simulink model "H8_2GDL_lineal_pruebas"  (R2022b)
settings: Solver=VariableStepAuto  StartTime=0.0  StopTime=5  RelTol=1e-3
InitFcn:
  | load("hems.mat");
  | airgap = hems.Airgap;
  | current = hems.Current;
  | forceV = hems.Force_Vertical;
  | forceH = hems.Force_Horizontal;
  | inductance = hems.Inductance;
  | resistance = hems.Resistance;
  | 
  | m = 200;
  | g = 9.81;
  | Iyy = 26.887;
  | x_lev12 = 0.443;
  | x_lev34 = 0.542;
  | z_max = 0.0225;
  | z_min = 0.01;
  | z_nom = 0.01965;
  | I_max = 50;
  | I_min = -50;
  | 
  | suelo = 0.0225;
  | techo = 0.01;
  | lev_nom = 0.01965;
  | time_stp = 2;
values from neighbouring files (symbols this model uses):
  A2 = argout.a    [linealizacion_2gdl.m]    (also in matrices_lineal_2gdl.mat = [0 0 689.948845287 37.4788996561 0 0 139.394129714 757.14948)
  B2 = argout.b    [linealizacion_2gdl.m]    (also in matrices_lineal_2gdl.mat = [0  0; 0  0; 0.151630617985  -0.185516467151; -0.09202917439)
  C2 = argout.c    [linealizacion_2gdl.m]    (also in matrices_lineal_2gdl.mat = [1 0 0 0 0 1 0 0 0 0 1 0 ... (16 elements, 4x4)])
  D2 = argout.d    [linealizacion_2gdl.m]    (also in matrices_lineal_2gdl.mat = [0  0; 0  0; 0  0; 0  0])
  Ka = [2091.38390024  -4523.40229407  65.4441805385  -70.1021906971  152.84626499  -886.851041867; -2276.61485995  -4503.65754193  -11.1725652788  -71.2004310761  -295.543801408  -714.324235622]    [Ka.mat]    (also in linealizacion_2gdl.m = place(Aa,Ba,[-5 -4 -6+6j -6-6j -2+2j -2-2j]))
undefined symbols (not defined in the file or in its folder): hems
libraries: slpidlib x4
settings Model: Creator=USUARIO  LastModifiedBy=ramuj

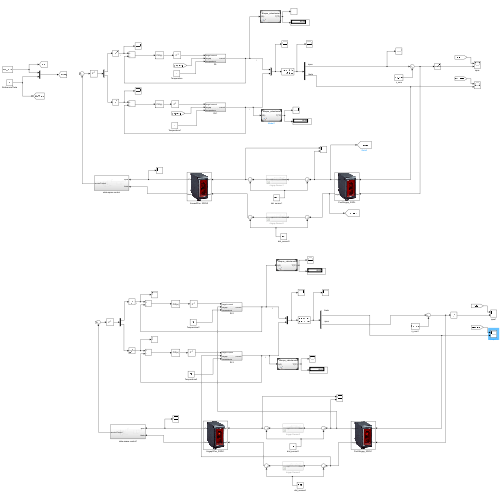
[thumbnail: Simulink's stored preview of the top-level diagram]
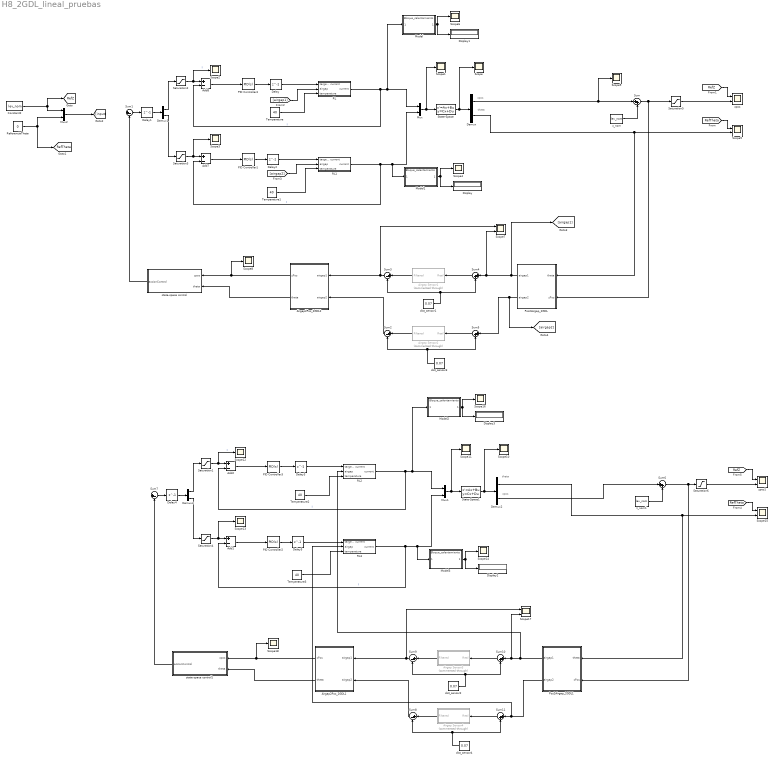
== system H8_2GDL_lineal_pruebas ==
  note: theta
  note: zpos
  note: zpos
  note: theta
  Add{1..2,7..8} (4 alike) : Sum  Inputs=+-
  Airgap Sensor1 : Subsystem  Commented=through
  Airgap Sensor2 : Subsystem  Commented=through
  Airgap Sensor3 : Subsystem  Commented=through
  Airgap Sensor4 : Subsystem  Commented=through
  Airgap2Pos_2GDL1 : Subsystem
      mask Display: image('C:\Users\ramuj\Desktop\Hyperloop\H8\Levitation-Repository\Levitation-Control-Dynamics\Modelo H8\image_airgapSensor.png'); % Use "Edit Image" on toolstrip to change.
  Airgap2Pos_2GDL2 : Subsystem
      mask Display: image('C:\Users\ramuj\Desktop\Hyperloop\H8\Levitation-Repository\Levitation-Control-Dynamics\Modelo H8\image_airgapSensor.png'); % Use "Edit Image" on toolstrip to change.
  Constant2 : Constant  Value=lev_nom
  Delay{,2..3,5} (4 alike) : Delay  DelayLength=1  SampleTime=1/(5e3)
  Delay1 : Delay  DelayLength=1  SampleTime=1/(1e3)
  Delay4 : Delay  DelayLength=1  SampleTime=1/(1e3)
  Demux{,1..3} (4 alike) : Demux  Outputs=2
  Display{,1..3} (4 alike) : Display
  Model{,1..3} (4 alike) : ModelReference  ModelNameDialog=Bloque_calentamiento.slx  SimulationMode=Normal  ModelReferenceVersion=3.3
  Mux : Mux  Inputs=2
  Mux1 : Mux  Inputs=2
  Mux2 : Mux  Inputs=2
  PID Controller{1..4} (4 alike) : slpidlib/PID Controller  Controller=PID  Form=Parallel  TimeDomain=Continuous-time  UseExternalTs=off  SampleTime=-1  IntegratorMethod=Forward Euler  FilterMethod=Forward Euler  ControllerParametersSource=internal  P=50  I=400  UseKiTs=off  D=0  N=0  UseFilter=on  TunerSelectOption=Transfer Function Based (PID Tuner App)  InitialConditionSource=internal  InitialConditionForIntegrator=0  InitialConditionForFilter=0  DifferentiatorICPrevScaledInput=0  ExternalReset=none  TrackingMode=off  Kt=1  LimitOutput=off  SatLimitsSource=internal  UpperSaturationLimit=inf  LowerSaturationLimit=-inf  LinearizeAsGain=on  AntiWindupMode=none  Kb=1  LimitIntegrator=off  UpperIntegratorSaturationLimit=inf  LowerIntegratorSaturationLimit=-inf  POutMin=[]  POutMax=[]  IOutMin=[]  IOutMax=[]  DOutMin=[]  DOutMax=[]  NOutMin=[]  NOutMax=[]  SumOutMin=[]  SumOutMax=[]  SaturationOutMin=[]  SaturationOutMax=[]  PParamMin=[]  PParamMax=[]  IParamMin=[]  IParamMax=[]  DParamMin=[]  DParamMax=[]  NParamMin=[]  NParamMax=[]  KbParamMin=[]  KbParamMax=[]  KtParamMin=[]  KtParamMax=[]  KbOutMin=[]  KbOutMax=[]  KtOutMin=[]  KtOutMax=[]  IntegratorOutMin=[]  IntegratorOutMax=[]  FilterOutMin=[]  FilterOutMax=[]  SumI1OutMin=[]  SumI1OutMax=[]  SumI2OutMin=[]  SumI2OutMax=[]  SumI3OutMin=[]  SumI3OutMax=[]  SumI4OutMin=[]  SumI4OutMax=[]  SumDOutMin=[]  SumDOutMax=[]  DifferentiatorOutMin=[]  DifferentiatorOutMax=[]  FilterDiffOutCoefMin=[]  FilterDiffOutCoefMax=[]  ReciprocalOutMin=[]  ReciprocalOutMax=[]  SumDenOutMin=[]  SumDenOutMax=[]  SumNumOutMin=[]  SumNumOutMax=[]  DivideOutMin=[]  DivideOutMax=[]  UdiffTsProdOutMin=[]  UdiffTsProdOutMax=[]  NTsProdOutMin=[]  NTsProdOutMax=[]  UintegralTsProdOutMin=[]  UintegralTsProdOutMax=[]  UngainTsProdOutMin=[]  UngainTsProdOutMax=[]  ClampingZeroOutDataTypeStr=Inherit: Inherit via back propagation  ClampingZeroOutMin=[]  ClampingZeroOutMax=[]  FilterDenConstantOutDataTypeStr=Inherit: Inherit via back propagation  FilterDenConstantOutMin=[]  FilterDenConstantOutMax=[]  PCopyOutDataTypeStr=Inherit: Inherit via back propagation  PCopyOutMin=[]  PCopyOutMax=[]  NCopyOutDataTypeStr=Inherit: Inherit via back propagation  NCopyOutMin=[]  NCopyOutMax=[]  IntegratorContinuousStateAttributes=''  IntegratorStateMustResolveToSignalObject=off  IntegratorRTWStateStorageClass=Auto  FilterContinuousStateAttributes=''  FilterStateMustResolveToSignalObject=off  FilterRTWStateStorageClass=Auto  ParallelPVariant=InternalParameters  IdealPVariant=Disabled  IVariant=InternalParameters  DVariant=InternalParameters  IntegratorVariant=Continuous  SatVariant=Disabled  AWVariant=Passthrough  PCopyVariant=Disabled  TRVariant=Disabled  FdbkBlocksVariant=Forward  IdealPFdbkVariant=Disabled  SatFdbkVariant=Disabled  DerivativeFilterVariant=ContFilter  NVariant=InternalParameters  NCopyVariant=Disabled  FilterICVariant=InternalICsFilter  IntegratorICVariant=InternalICs  ExternalResetVariant=Disabled  TRSumVariant=Passthrough  SumFdbkVariant=Disabled  SumVariant=Sum_PID  TsampFilterVariant=InternalTs  TsampNgainVariant=Passthrough  TsampIntegralVariant=Passthrough  ExternalSaturationOutDataTypeStr=Inherit: Same as second input
  Pos2Airgap_2GDL : Subsystem
      mask Display: image('C:\Users\ramuj\Desktop\Hyperloop\H8\Levitation-Repository\Levitation-Control-Dynamics\Modelo H8\image_airgapSensor.png'); % Use "Edit Image" on toolstrip to change.
  Pos2Airgap_2GDL1 : Subsystem
      mask Display: image('C:\Users\ramuj\Desktop\Hyperloop\H8\Levitation-Repository\Levitation-Control-Dynamics\Modelo H8\image_airgapSensor.png'); % Use "Edit Image" on toolstrip to change.
  RL : Subsystem
  RL1 : Subsystem
  RL2 : Subsystem
  RL3 : Subsystem
  ReferenciaTheta : Constant  Value=0
  Saturation{1..4} (4 alike) : Saturate  UpperLimit=I_max  LowerLimit=I_min
  Saturation5 : Saturate  UpperLimit=suelo  LowerLimit=techo
  Saturation6 : Saturate  UpperLimit=suelo  LowerLimit=techo
  Scope{,1..4,6,8..14,16,18} (15 alike) : Scope
  Scope{5,7,15,17} (4 alike) : Scope  NumInputPorts=2
  State-Space : StateSpace  A=A2  B=B2  C=C2  D=D2  InitialCondition=[0, suelo-lev_nom, 0, 0]
  State-Space1 : StateSpace  A=A2  B=B2  C=C2  D=D2  InitialCondition=[0, suelo-lev_nom, 0, 0]
  Sum{,4..6,10..11} (6 alike) : Sum  Inputs=|++
  Sum{1..3,7..9} (6 alike) : Sum  Inputs=|+-
  Temperature{,1..3} (4 alike) : Constant  Value=40
  dist_sensor{1..4} (4 alike) : Constant  Value=0.07
  state-space control : Subsystem
  state-space control1 : Subsystem
  z_nom : Constant  Value=lev_nom
  z_nom1 : Constant  Value=lev_nom
  zpos : Scope  NumInputPorts=2
  zpos1 : Scope  NumInputPorts=2
  tag scope: RefTheta=global, RefZ=global
  wires:
  PID Controller1/1 -> Delay2/1
  Saturation3/1 -> Scope3/1, Add7/1
  RL/1(current) -> Add8/2, Model/1, Mux/1  "I"
  PID Controller4/1 -> Delay/1
  Saturation2/1 -> Scope2/1, Add8/1  "I"
  State-Space/1 -> Demux/1, Scope/1
  Mux/1 -> Scope1/1, State-Space/1
  RL1/1(current) -> Add7/2, Mux/2, Model1/1  "I"
  z_nom/1 -> Sum/2
  Temperature/1 -> RL/3(temperature)
  Temperature1/1 -> RL1/3(temperature)
  Constant2/1 -> [RefZ], Mux2/1
  ReferenciaTheta/1 -> Mux2/2, [RefTheta]
  Mux2/1 -> [input]
  Demux1/1 -> Saturation2/1
  Demux1/2 -> Saturation3/1
  [RefTheta] -> Scope5/1
  [RefZ] -> zpos/1
  Add8/1 -> PID Controller4/1
  Add7/1 -> PID Controller1/1
  Sum1/1 -> Delay1/1
  Saturation5/1 -> zpos/2
  Model1/1 -> Scope4/1, Display/1
  Model/1 -> Scope6/1, Display1/1
  Demux/1 -> Sum/1, Scope9/1
  state-space control/1(accionControl) -> Sum1/2
  Delay1/1 -> Demux1/1
  Delay/1 -> RL/1(target current)
  Delay2/1 -> RL1/1(target current)
  Sum/1 -> Pos2Airgap_2GDL/2(zPos), Saturation5/1
  Airgap2Pos_2GDL2/1(zPos) -> Scope8/1, state-space control/1(zpos)
  Airgap2Pos_2GDL2/2(theta) -> state-space control/2(theta)
  dist_sensor1/1 -> Sum4/2, Sum3/2
  Airgap Sensor1/1(Filtered) -> Sum3/1
  Sum4/1 -> Airgap Sensor1/1(Real)
  Sum3/1 -> Scope7/1, Airgap2Pos_2GDL2/1(airgap1)
  Pos2Airgap_2GDL/1(airgap1) -> Scope7/2, Sum4/1, [airgap1]
  dist_sensor3/1 -> Sum5/2, Sum2/2
  Airgap Sensor2/1(Filtered) -> Sum2/1
  Sum5/1 -> Airgap Sensor2/1(Real)
  Pos2Airgap_2GDL/2(airgap2) -> [airgap2], Sum5/1
  Sum2/1 -> Airgap2Pos_2GDL2/2(airgap2)
  [airgap1] -> RL/2(airgap)
  [airgap2] -> RL1/2(airgap)
  Demux/2 -> Pos2Airgap_2GDL/1(theta), Scope5/2
  state-space control1/1(accionControl) -> Sum7/2
  Pos2Airgap_2GDL1/1(airgap1) -> RL2/2(airgap), Scope17/2, Sum10/1
  dist_sensor2/1 -> Sum10/2, Sum9/2
  Sum10/1 -> Airgap Sensor3/1(Real)
  Pos2Airgap_2GDL1/2(airgap2) -> RL3/2(airgap), Sum11/1
  Airgap Sensor3/1(Filtered) -> Sum9/1
  Sum6/1 -> Pos2Airgap_2GDL1/2(zPos), Saturation6/1
  Airgap2Pos_2GDL1/2(theta) -> state-space control1/2(theta)
  Sum11/1 -> Airgap Sensor4/1(Real)
  Airgap Sensor4/1(Filtered) -> Sum8/1
  dist_sensor4/1 -> Sum11/2, Sum8/2
  PID Controller2/1 -> Delay5/1
  State-Space1/1 -> Demux2/1, Scope10/1
  Temperature3/1 -> RL3/3(temperature)
  Model2/1 -> Scope16/1, Display3/1
  Demux3/2 -> Saturation4/1
  Delay3/1 -> RL2/1(target current)
  Saturation4/1 -> Scope13/1, Add1/1
  Model3/1 -> Scope14/1, Display2/1
  Delay5/1 -> RL3/1(target current)
  Sum8/1 -> Airgap2Pos_2GDL1/2(airgap2)
  Saturation6/1 -> zpos1/2
  RL2/1(current) -> Add2/2, Model2/1, Mux1/1  "I"
  Airgap2Pos_2GDL1/1(zPos) -> Scope18/1, state-space control1/1(zpos)
  Temperature2/1 -> RL2/3(temperature)
  [RefZ] -> zpos1/1
  Sum7/1 -> Delay4/1
  [RefTheta] -> Scope15/1
  Demux3/1 -> Saturation1/1
  Add2/1 -> PID Controller3/1
  Add1/1 -> PID Controller2/1
  Saturation1/1 -> Scope12/1, Add2/1  "I"
  PID Controller3/1 -> Delay3/1
  z_nom1/1 -> Sum6/2
  RL3/1(current) -> Add1/2, Mux1/2, Model3/1  "I"
  Delay4/1 -> Demux3/1
  Sum9/1 -> Scope17/1, Airgap2Pos_2GDL1/1(airgap1)
  Mux1/1 -> Scope11/1, State-Space1/1
  Demux2/1 -> Pos2Airgap_2GDL1/1(theta), Scope15/2
  Demux2/2 -> Sum6/1

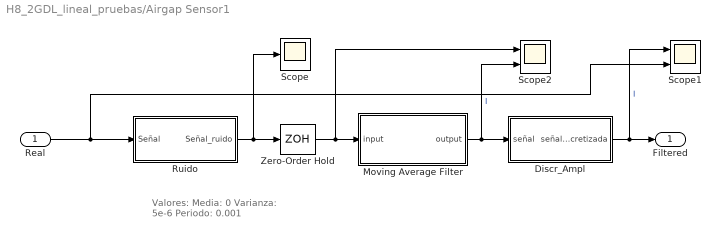
== system H8_2GDL_lineal_pruebas/Airgap Sensor1 ==
  note: Valores:
      | Media: 0
      | Varianza: 5e-6
      | Periodo: 0.001
  Real : Inport
  Discr_Ampl : Subsystem  mask{N=1024, Min=0.065, Max=0.105}
      mask prompts: N "Valores distintos (N)"; Min "Valor mínimo"; Max "Valor máximo"
      mask DialogControl DescGroupVar Prompt: Discretizacion_Amplitud
      mask DialogControl DescTextVar Prompt: Discretización en amplitud
  Moving Average Filter : Subsystem  mask{M=2, fs=-1}
      mask prompts: M "Orden del filtro (M)"; fs "Frecuencia de muestreo (fs)"
  Ruido : Subsystem  mask{M=0, V=5e-8, T=0.001}
      mask prompts: M "Media"; V "Varianza"; T "Periodo"
      mask DialogControl Ruido Prompt: Ruido
      mask DialogControl DescTextVar Prompt: Añade ruido gaussiano
  Scope : Scope
  Scope1 : Scope  NumInputPorts=2
  Scope2 : Scope  NumInputPorts=2
  Zero-Order Hold : ZeroOrderHold  SampleTime=1/(1*10^3)
  Filtered : Outport
  wires:
  Real/1 -> Scope1/2, Ruido/1(Señal)
  Discr_Ampl/1(señal_discretizada) -> Scope1/1, Filtered/1  "I"
  Moving Average Filter/1(output) -> Scope2/2, Discr_Ampl/1(señal)  "I"
  Ruido/1(Señal_ruido) -> Scope/1, Zero-Order Hold/1
  Zero-Order Hold/1 -> Moving Average Filter/1(input), Scope2/1

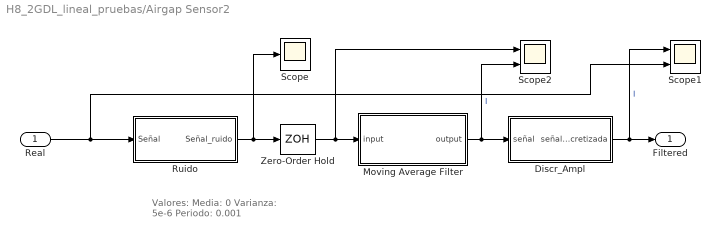
== system H8_2GDL_lineal_pruebas/Airgap Sensor2 ==
  note: Valores:
      | Media: 0
      | Varianza: 5e-6
      | Periodo: 0.001
  Real : Inport
  Discr_Ampl : Subsystem  mask{N=1024, Min=0.065, Max=0.105}
      mask prompts: N "Valores distintos (N)"; Min "Valor mínimo"; Max "Valor máximo"
      mask DialogControl DescGroupVar Prompt: Discretizacion_Amplitud
      mask DialogControl DescTextVar Prompt: Discretización en amplitud
  Moving Average Filter : Subsystem  mask{M=2, fs=-1}
      mask prompts: M "Orden del filtro (M)"; fs "Frecuencia de muestreo (fs)"
  Ruido : Subsystem  mask{M=0, V=5e-8, T=0.001}
      mask prompts: M "Media"; V "Varianza"; T "Periodo"
      mask DialogControl Ruido Prompt: Ruido
      mask DialogControl DescTextVar Prompt: Añade ruido gaussiano
  Scope : Scope
  Scope1 : Scope  NumInputPorts=2
  Scope2 : Scope  NumInputPorts=2
  Zero-Order Hold : ZeroOrderHold  SampleTime=1/(1*10^3)
  Filtered : Outport
  wires:
  Real/1 -> Scope1/2, Ruido/1(Señal)
  Discr_Ampl/1(señal_discretizada) -> Scope1/1, Filtered/1  "I"
  Moving Average Filter/1(output) -> Scope2/2, Discr_Ampl/1(señal)  "I"
  Ruido/1(Señal_ruido) -> Scope/1, Zero-Order Hold/1
  Zero-Order Hold/1 -> Moving Average Filter/1(input), Scope2/1

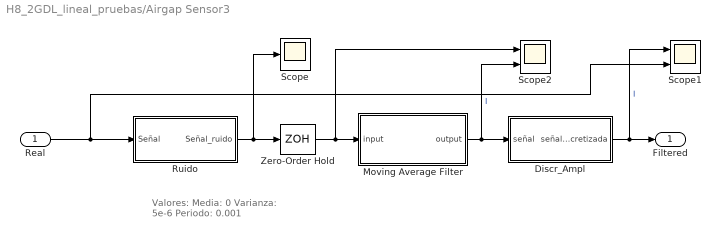
== system H8_2GDL_lineal_pruebas/Airgap Sensor3 ==
  note: Valores:
      | Media: 0
      | Varianza: 5e-6
      | Periodo: 0.001
  Real : Inport
  Discr_Ampl : Subsystem  mask{N=1024, Min=0.065, Max=0.105}
      mask prompts: N "Valores distintos (N)"; Min "Valor mínimo"; Max "Valor máximo"
      mask DialogControl DescGroupVar Prompt: Discretizacion_Amplitud
      mask DialogControl DescTextVar Prompt: Discretización en amplitud
  Moving Average Filter : Subsystem  mask{M=2, fs=-1}
      mask prompts: M "Orden del filtro (M)"; fs "Frecuencia de muestreo (fs)"
  Ruido : Subsystem  mask{M=0, V=5e-8, T=0.001}
      mask prompts: M "Media"; V "Varianza"; T "Periodo"
      mask DialogControl Ruido Prompt: Ruido
      mask DialogControl DescTextVar Prompt: Añade ruido gaussiano
  Scope : Scope
  Scope1 : Scope  NumInputPorts=2
  Scope2 : Scope  NumInputPorts=2
  Zero-Order Hold : ZeroOrderHold  SampleTime=1/(1*10^3)
  Filtered : Outport
  wires:
  Real/1 -> Scope1/2, Ruido/1(Señal)
  Discr_Ampl/1(señal_discretizada) -> Scope1/1, Filtered/1  "I"
  Moving Average Filter/1(output) -> Scope2/2, Discr_Ampl/1(señal)  "I"
  Ruido/1(Señal_ruido) -> Scope/1, Zero-Order Hold/1
  Zero-Order Hold/1 -> Moving Average Filter/1(input), Scope2/1

== system H8_2GDL_lineal_pruebas/Airgap Sensor4 ==
  note: Valores:
      | Media: 0
      | Varianza: 5e-6
      | Periodo: 0.001
  Real : Inport
  Discr_Ampl : Subsystem  mask{N=1024, Min=0.065, Max=0.105}
      mask prompts: N "Valores distintos (N)"; Min "Valor mínimo"; Max "Valor máximo"
      mask DialogControl DescGroupVar Prompt: Discretizacion_Amplitud
      mask DialogControl DescTextVar Prompt: Discretización en amplitud
  Moving Average Filter : Subsystem  mask{M=2, fs=-1}
      mask prompts: M "Orden del filtro (M)"; fs "Frecuencia de muestreo (fs)"
  Ruido : Subsystem  mask{M=0, V=5e-8, T=0.001}
      mask prompts: M "Media"; V "Varianza"; T "Periodo"
      mask DialogControl Ruido Prompt: Ruido
      mask DialogControl DescTextVar Prompt: Añade ruido gaussiano
  Scope : Scope
  Scope1 : Scope  NumInputPorts=2
  Scope2 : Scope  NumInputPorts=2
  Zero-Order Hold : ZeroOrderHold  SampleTime=1/(1*10^3)
  Filtered : Outport
  wires:
  Real/1 -> Scope1/2, Ruido/1(Señal)
  Discr_Ampl/1(señal_discretizada) -> Scope1/1, Filtered/1  "I"
  Moving Average Filter/1(output) -> Scope2/2, Discr_Ampl/1(señal)  "I"
  Ruido/1(Señal_ruido) -> Scope/1, Zero-Order Hold/1
  Zero-Order Hold/1 -> Moving Average Filter/1(input), Scope2/1

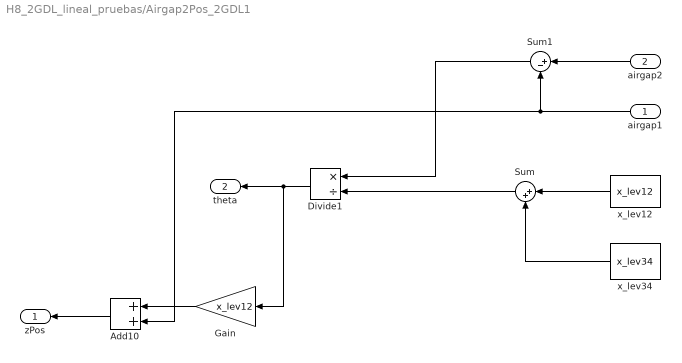
== system H8_2GDL_lineal_pruebas/Airgap2Pos_2GDL1 ==
  airgap1 : Inport
  airgap2 : Inport  Port=2
  Add10 : Sum
  Divide1 : Product  Inputs=*/
  Gain : Gain  Gain=x_lev12
  Sum : Sum  Inputs=|++
  Sum1 : Sum  Inputs=|+-
  x_lev12 : Constant  Value=x_lev12
  x_lev34 : Constant  Value=x_lev34
  zPos : Outport
  theta : Outport  Port=2
  wires:
  Add10/1 -> zPos/1
  Divide1/1 -> theta/1, Gain/1
  x_lev12/1 -> Sum/1
  x_lev34/1 -> Sum/2
  Sum/1 -> Divide1/2
  airgap2/1 -> Sum1/1
  airgap1/1 -> Sum1/2, Add10/2
  Sum1/1 -> Divide1/1
  Gain/1 -> Add10/1

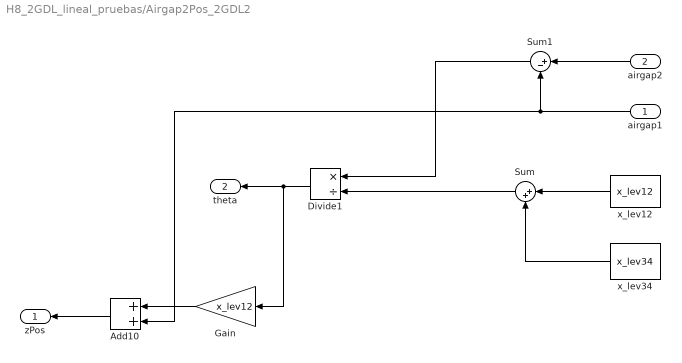
== system H8_2GDL_lineal_pruebas/Airgap2Pos_2GDL2 ==
  airgap1 : Inport
  airgap2 : Inport  Port=2
  Add10 : Sum
  Divide1 : Product  Inputs=*/
  Gain : Gain  Gain=x_lev12
  Sum : Sum  Inputs=|++
  Sum1 : Sum  Inputs=|+-
  x_lev12 : Constant  Value=x_lev12
  x_lev34 : Constant  Value=x_lev34
  zPos : Outport
  theta : Outport  Port=2
  wires:
  Add10/1 -> zPos/1
  Divide1/1 -> theta/1, Gain/1
  x_lev12/1 -> Sum/1
  x_lev34/1 -> Sum/2
  Sum/1 -> Divide1/2
  airgap2/1 -> Sum1/1
  airgap1/1 -> Sum1/2, Add10/2
  Sum1/1 -> Divide1/1
  Gain/1 -> Add10/1

== system H8_2GDL_lineal_pruebas/Pos2Airgap_2GDL ==
  theta : Inport
  zPos : Inport  Port=2
  Add10 : Sum
  Add11 : Sum  Inputs=-+
  Gain3 : Gain  Gain=x_lev12
  Gain4 : Gain  Gain=x_lev34
  airgap1 : Outport
  airgap2 : Outport  Port=2
  wires:
  Add10/1 -> airgap2/1
  zPos/1 -> Add11/2, Add10/2
  theta/1 -> Gain4/1, Gain3/1
  Gain3/1 -> Add11/1
  Gain4/1 -> Add10/1
  Add11/1 -> airgap1/1

== system H8_2GDL_lineal_pruebas/Pos2Airgap_2GDL1 ==
  theta : Inport
  zPos : Inport  Port=2
  Add10 : Sum
  Add11 : Sum  Inputs=-+
  Gain3 : Gain  Gain=x_lev12
  Gain4 : Gain  Gain=x_lev34
  airgap1 : Outport
  airgap2 : Outport  Port=2
  wires:
  Add10/1 -> airgap2/1
  zPos/1 -> Add11/2, Add10/2
  theta/1 -> Gain4/1, Gain3/1
  Gain3/1 -> Add11/1
  Gain4/1 -> Add10/1
  Add11/1 -> airgap1/1

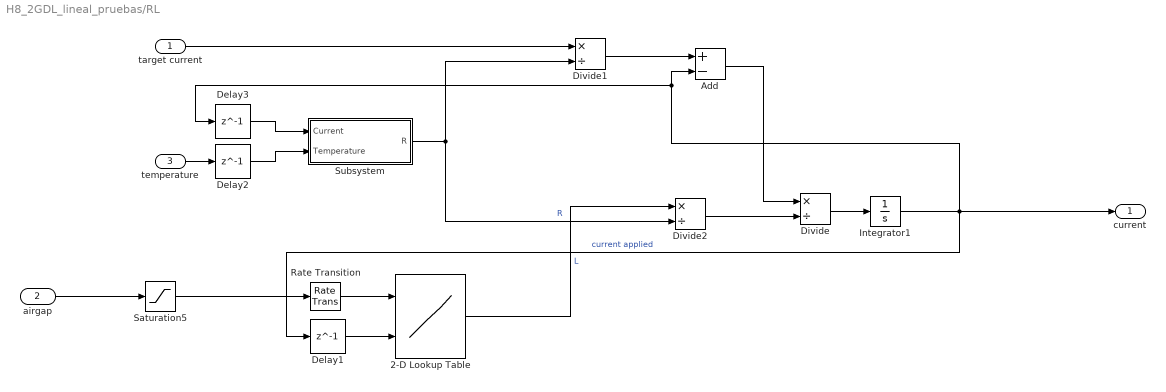
== system H8_2GDL_lineal_pruebas/RL ==
  target current : Inport
  airgap : Inport  Port=2
  temperature : Inport  Port=3
  2-D Lookup Table : Lookup_n-D  BreakpointsForDimension1=hems.Airgap  BreakpointsForDimension2=hems.Current(2:110)  Table=hems.Inductance  InternalRulePriority=Speed  RndMeth=Simplest
      settings: InputPortMap=u0,u1
  Add : Sum  Inputs=+-
  Delay1 : Delay  DelayLength=1
  Delay2 : Delay  DelayLength=1
  Delay3 : Delay  DelayLength=1
  Divide : Product  Inputs=*/
  Divide1 : Product  Inputs=*/
  Divide2 : Product  Inputs=*/
  Integrator1 : Integrator
  Rate Transition : RateTransition
  Saturation5 : Saturate  UpperLimit=suelo  LowerLimit=techo
  Subsystem : Subsystem
  current : Outport
  wires:
  airgap/1 -> Saturation5/1
  Divide/1 -> Integrator1/1
  Add/1 -> Divide/1
  Integrator1/1 -> Delay1/1, current/1, Delay3/1, Add/2  "current applied"
  2-D Lookup Table/1 -> Divide2/1  "L"
  target current/1 -> Divide1/1
  temperature/1 -> Delay2/1
  Divide1/1 -> Add/1
  Subsystem/1(R) -> Divide2/2, Divide1/2  "R"
  Delay3/1 -> Subsystem/1(Current)
  Delay2/1 -> Subsystem/2(Temperature)
  Divide2/1 -> Divide/2
  Delay1/1 -> 2-D Lookup Table/2
  Rate Transition/1 -> 2-D Lookup Table/1
  Saturation5/1 -> Rate Transition/1

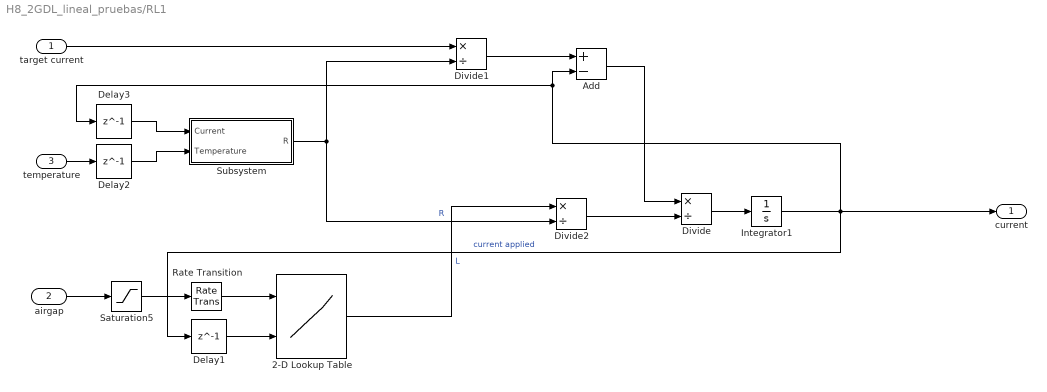
== system H8_2GDL_lineal_pruebas/RL1 ==
  target current : Inport
  airgap : Inport  Port=2
  temperature : Inport  Port=3
  2-D Lookup Table : Lookup_n-D  BreakpointsForDimension1=hems.Airgap  BreakpointsForDimension2=hems.Current(2:110)  Table=hems.Inductance  InternalRulePriority=Speed  RndMeth=Simplest
      settings: InputPortMap=u0,u1
  Add : Sum  Inputs=+-
  Delay1 : Delay  DelayLength=1
  Delay2 : Delay  DelayLength=1
  Delay3 : Delay  DelayLength=1
  Divide : Product  Inputs=*/
  Divide1 : Product  Inputs=*/
  Divide2 : Product  Inputs=*/
  Integrator1 : Integrator
  Rate Transition : RateTransition
  Saturation5 : Saturate  UpperLimit=suelo  LowerLimit=techo
  Subsystem : Subsystem
  current : Outport
  wires:
  airgap/1 -> Saturation5/1
  Divide/1 -> Integrator1/1
  Add/1 -> Divide/1
  Integrator1/1 -> Delay1/1, current/1, Delay3/1, Add/2  "current applied"
  2-D Lookup Table/1 -> Divide2/1  "L"
  target current/1 -> Divide1/1
  temperature/1 -> Delay2/1
  Divide1/1 -> Add/1
  Subsystem/1(R) -> Divide2/2, Divide1/2  "R"
  Delay3/1 -> Subsystem/1(Current)
  Delay2/1 -> Subsystem/2(Temperature)
  Divide2/1 -> Divide/2
  Delay1/1 -> 2-D Lookup Table/2
  Rate Transition/1 -> 2-D Lookup Table/1
  Saturation5/1 -> Rate Transition/1

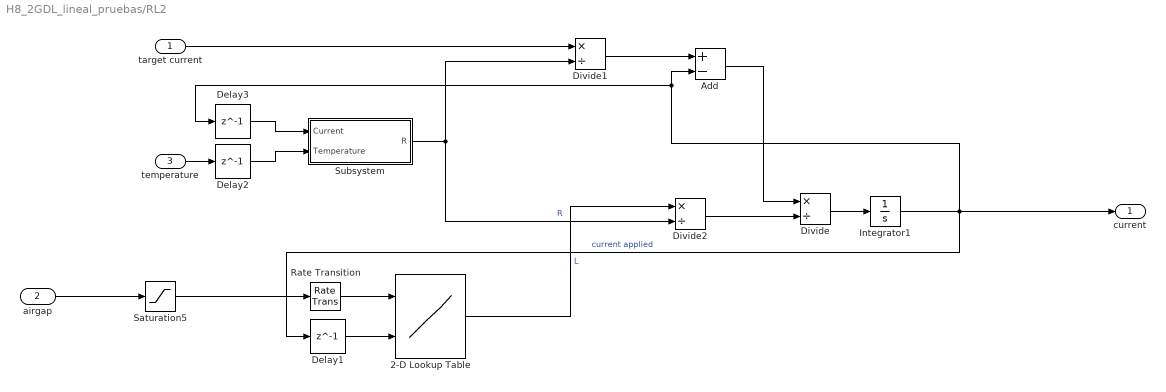
== system H8_2GDL_lineal_pruebas/RL2 ==
  target current : Inport
  airgap : Inport  Port=2
  temperature : Inport  Port=3
  2-D Lookup Table : Lookup_n-D  BreakpointsForDimension1=hems.Airgap  BreakpointsForDimension2=hems.Current(2:110)  Table=hems.Inductance  InternalRulePriority=Speed  RndMeth=Simplest
      settings: InputPortMap=u0,u1
  Add : Sum  Inputs=+-
  Delay1 : Delay  DelayLength=1
  Delay2 : Delay  DelayLength=1
  Delay3 : Delay  DelayLength=1
  Divide : Product  Inputs=*/
  Divide1 : Product  Inputs=*/
  Divide2 : Product  Inputs=*/
  Integrator1 : Integrator
  Rate Transition : RateTransition
  Saturation5 : Saturate  UpperLimit=suelo  LowerLimit=techo
  Subsystem : Subsystem
  current : Outport
  wires:
  airgap/1 -> Saturation5/1
  Divide/1 -> Integrator1/1
  Add/1 -> Divide/1
  Integrator1/1 -> Delay1/1, current/1, Delay3/1, Add/2  "current applied"
  2-D Lookup Table/1 -> Divide2/1  "L"
  target current/1 -> Divide1/1
  temperature/1 -> Delay2/1
  Divide1/1 -> Add/1
  Subsystem/1(R) -> Divide2/2, Divide1/2  "R"
  Delay3/1 -> Subsystem/1(Current)
  Delay2/1 -> Subsystem/2(Temperature)
  Divide2/1 -> Divide/2
  Delay1/1 -> 2-D Lookup Table/2
  Rate Transition/1 -> 2-D Lookup Table/1
  Saturation5/1 -> Rate Transition/1

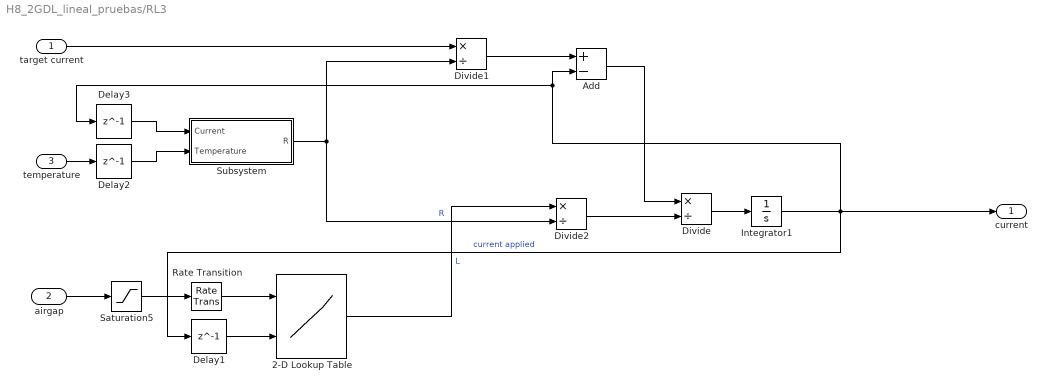
== system H8_2GDL_lineal_pruebas/RL3 ==
  target current : Inport
  airgap : Inport  Port=2
  temperature : Inport  Port=3
  2-D Lookup Table : Lookup_n-D  BreakpointsForDimension1=hems.Airgap  BreakpointsForDimension2=hems.Current(2:110)  Table=hems.Inductance  InternalRulePriority=Speed  RndMeth=Simplest
      settings: InputPortMap=u0,u1
  Add : Sum  Inputs=+-
  Delay1 : Delay  DelayLength=1
  Delay2 : Delay  DelayLength=1
  Delay3 : Delay  DelayLength=1
  Divide : Product  Inputs=*/
  Divide1 : Product  Inputs=*/
  Divide2 : Product  Inputs=*/
  Integrator1 : Integrator
  Rate Transition : RateTransition
  Saturation5 : Saturate  UpperLimit=suelo  LowerLimit=techo
  Subsystem : Subsystem
  current : Outport
  wires:
  airgap/1 -> Saturation5/1
  Divide/1 -> Integrator1/1
  Add/1 -> Divide/1
  Integrator1/1 -> Delay1/1, current/1, Delay3/1, Add/2  "current applied"
  2-D Lookup Table/1 -> Divide2/1  "L"
  target current/1 -> Divide1/1
  temperature/1 -> Delay2/1
  Divide1/1 -> Add/1
  Subsystem/1(R) -> Divide2/2, Divide1/2  "R"
  Delay3/1 -> Subsystem/1(Current)
  Delay2/1 -> Subsystem/2(Temperature)
  Divide2/1 -> Divide/2
  Delay1/1 -> 2-D Lookup Table/2
  Rate Transition/1 -> 2-D Lookup Table/1
  Saturation5/1 -> Rate Transition/1

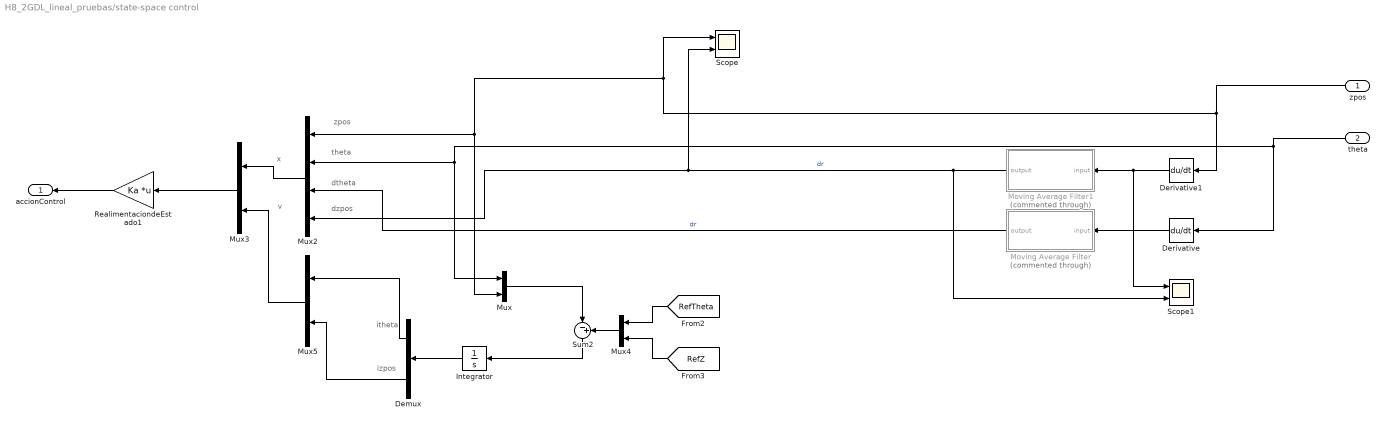
== system H8_2GDL_lineal_pruebas/state-space control ==
  note: itheta
  note: v
  note: x
  note: dtheta
  note: dzpos
  note: zpos
  note: theta
  note: izpos
  zpos : Inport
  theta : Inport  Port=2
  Demux : Demux  Outputs=2
  Derivative : Derivative
  Derivative1 : Derivative
  Integrator : Integrator
  Moving Average Filter : Subsystem  Commented=through  mask{M=2, fs=-1}
      mask prompts: M "Orden del filtro (M)"; fs "Frecuencia de muestreo (fs)"
  Moving Average Filter1 : Subsystem  Commented=through  mask{M=2, fs=-1}
      mask prompts: M "Orden del filtro (M)"; fs "Frecuencia de muestreo (fs)"
  Mux{,3..5} (4 alike) : Mux  Inputs=2
  Mux2 : Mux
  RealimentaciondeEstado1 : Gain  Gain=Ka  Multiplication=Matrix(K*u)
  Scope : Scope  NumInputPorts=2
  Scope1 : Scope  NumInputPorts=2
  Sum2 : Sum  Inputs=|-+
  accionControl : Outport
  wires:
  [RefZ] -> Mux4/2
  Derivative1/1 -> Scope1/1, Moving Average Filter1/1(input)
  zpos/1 -> Scope/1, Mux/2, Mux2/1, Derivative1/1
  Mux4/1 -> Sum2/2
  Sum2/1 -> Integrator/1
  Mux3/1 -> RealimentaciondeEstado1/1
  theta/1 -> Derivative/1, Mux2/2, Mux/1
  [RefTheta] -> Mux4/1
  Derivative/1 -> Moving Average Filter/1(input)
  RealimentaciondeEstado1/1 -> accionControl/1
  Mux/1 -> Sum2/1
  Moving Average Filter/1(output) -> Mux2/3  "dr"
  Moving Average Filter1/1(output) -> Scope1/2, Mux2/4, Scope/2  "dr"
  Mux5/1 -> Mux3/2
  Mux2/1 -> Mux3/1
  Integrator/1 -> Demux/1
  Demux/2 -> Mux5/2
  Demux/1 -> Mux5/1

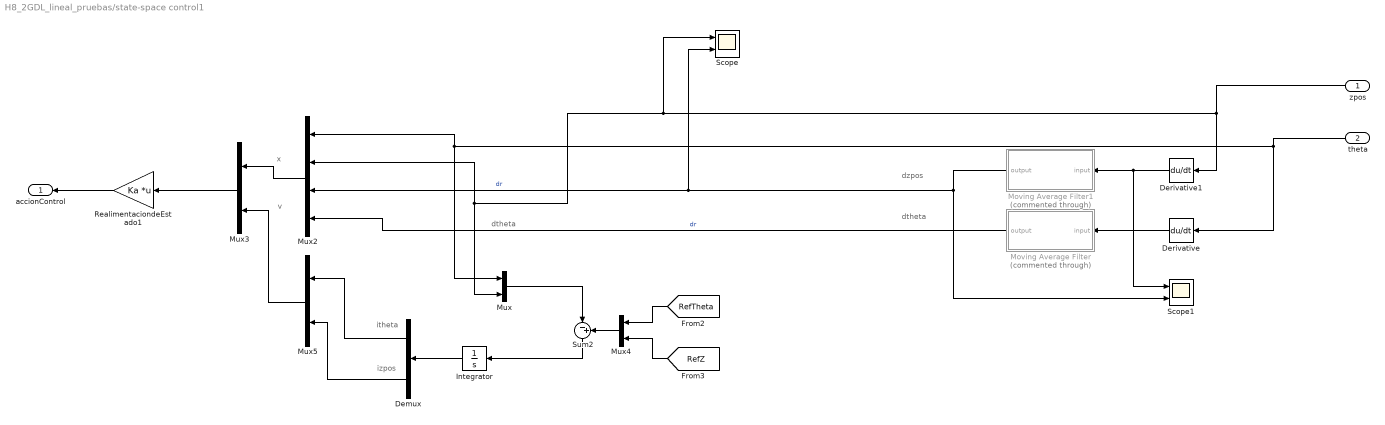
== system H8_2GDL_lineal_pruebas/state-space control1 ==
  note: dzpos
  note: itheta
  note: v
  note: x
  note: dtheta
  note: izpos
  note: dtheta
  zpos : Inport
  theta : Inport  Port=2
  Demux : Demux  Outputs=2
  Derivative : Derivative
  Derivative1 : Derivative
  Integrator : Integrator
  Moving Average Filter : Subsystem  Commented=through  mask{M=2, fs=-1}
      mask prompts: M "Orden del filtro (M)"; fs "Frecuencia de muestreo (fs)"
  Moving Average Filter1 : Subsystem  Commented=through  mask{M=2, fs=-1}
      mask prompts: M "Orden del filtro (M)"; fs "Frecuencia de muestreo (fs)"
  Mux{,3..5} (4 alike) : Mux  Inputs=2
  Mux2 : Mux
  RealimentaciondeEstado1 : Gain  Gain=Ka  Multiplication=Matrix(K*u)
  Scope : Scope  NumInputPorts=2
  Scope1 : Scope  NumInputPorts=2
  Sum2 : Sum  Inputs=|-+
  accionControl : Outport
  wires:
  [RefZ] -> Mux4/2
  Derivative1/1 -> Scope1/1, Moving Average Filter1/1(input)
  zpos/1 -> Scope/1, Mux2/2, Mux/2, Derivative1/1
  Mux4/1 -> Sum2/2
  Sum2/1 -> Integrator/1
  Mux3/1 -> RealimentaciondeEstado1/1
  theta/1 -> Derivative/1, Mux/1, Mux2/1
  [RefTheta] -> Mux4/1
  Derivative/1 -> Moving Average Filter/1(input)
  RealimentaciondeEstado1/1 -> accionControl/1
  Mux/1 -> Sum2/1
  Moving Average Filter/1(output) -> Mux2/4  "dr"
  Moving Average Filter1/1(output) -> Scope1/2, Scope/2, Mux2/3  "dr"
  Mux5/1 -> Mux3/2
  Mux2/1 -> Mux3/1
  Integrator/1 -> Demux/1
  Demux/2 -> Mux5/2
  Demux/1 -> Mux5/1

== system H8_2GDL_lineal_pruebas/Airgap Sensor1/Discr_Ampl ==
  señal : Inport
  Constant : Constant  Value=N
  Constant1 : Constant  Value=Max
  Constant2 : Constant  Value=Min
  MATLAB Function1 : MATLAB Function  TreatAsAtomicUnit=on
  señal_discretizada : Outport
  wires:
  MATLAB Function1/1(senal_discretizada) -> señal_discretizada/1
  señal/1 -> MATLAB Function1/1(senal)
  Constant1/1 -> MATLAB Function1/3(Max)
  Constant/1 -> MATLAB Function1/2(N)
  Constant2/1 -> MATLAB Function1/4(Min)

== system H8_2GDL_lineal_pruebas/Airgap Sensor1/Moving Average Filter ==
  input : Inport
  Delay : Delay  DelayLength=M  SampleTime=fs
  Delay1 : Delay  DelayLength=1  SampleTime=fs
  Gain : Gain  Gain=1/M
  Sum : Sum  Inputs=|+-
  Sum1 : Sum  Inputs=|++
  output : Outport
  wires:
  input/1 -> Delay/1, Sum/1
  Delay/1 -> Sum/2
  Sum/1 -> Sum1/1
  Sum1/1 -> Delay1/1, Gain/1
  Delay1/1 -> Sum1/2
  Gain/1 -> output/1

== system H8_2GDL_lineal_pruebas/Airgap Sensor1/Ruido ==
  Señal : Inport
  Random Number : RandomNumber  Mean=M  Variance=V  Seed=3  SampleTime=T
  Sum : Sum  Inputs=|++
  Señal_ruido : Outport
  wires:
  Random Number/1 -> Sum/2
  Señal/1 -> Sum/1
  Sum/1 -> Señal_ruido/1

== system H8_2GDL_lineal_pruebas/Airgap Sensor2/Discr_Ampl ==
  señal : Inport
  Constant : Constant  Value=N
  Constant1 : Constant  Value=Max
  Constant2 : Constant  Value=Min
  MATLAB Function1 : MATLAB Function  TreatAsAtomicUnit=on
  señal_discretizada : Outport
  wires:
  MATLAB Function1/1(senal_discretizada) -> señal_discretizada/1
  señal/1 -> MATLAB Function1/1(senal)
  Constant1/1 -> MATLAB Function1/3(Max)
  Constant/1 -> MATLAB Function1/2(N)
  Constant2/1 -> MATLAB Function1/4(Min)

== system H8_2GDL_lineal_pruebas/Airgap Sensor2/Moving Average Filter ==
  input : Inport
  Delay : Delay  DelayLength=M  SampleTime=fs
  Delay1 : Delay  DelayLength=1  SampleTime=fs
  Gain : Gain  Gain=1/M
  Sum : Sum  Inputs=|+-
  Sum1 : Sum  Inputs=|++
  output : Outport
  wires:
  input/1 -> Delay/1, Sum/1
  Delay/1 -> Sum/2
  Sum/1 -> Sum1/1
  Sum1/1 -> Delay1/1, Gain/1
  Delay1/1 -> Sum1/2
  Gain/1 -> output/1

== system H8_2GDL_lineal_pruebas/Airgap Sensor2/Ruido ==
  Señal : Inport
  Random Number : RandomNumber  Mean=M  Variance=V  Seed=3  SampleTime=T
  Sum : Sum  Inputs=|++
  Señal_ruido : Outport
  wires:
  Random Number/1 -> Sum/2
  Señal/1 -> Sum/1
  Sum/1 -> Señal_ruido/1

== system H8_2GDL_lineal_pruebas/Airgap Sensor3/Discr_Ampl ==
  señal : Inport
  Constant : Constant  Value=N
  Constant1 : Constant  Value=Max
  Constant2 : Constant  Value=Min
  MATLAB Function1 : MATLAB Function  TreatAsAtomicUnit=on
  señal_discretizada : Outport
  wires:
  MATLAB Function1/1(senal_discretizada) -> señal_discretizada/1
  señal/1 -> MATLAB Function1/1(senal)
  Constant1/1 -> MATLAB Function1/3(Max)
  Constant/1 -> MATLAB Function1/2(N)
  Constant2/1 -> MATLAB Function1/4(Min)

== system H8_2GDL_lineal_pruebas/Airgap Sensor3/Moving Average Filter ==
  input : Inport
  Delay : Delay  DelayLength=M  SampleTime=fs
  Delay1 : Delay  DelayLength=1  SampleTime=fs
  Gain : Gain  Gain=1/M
  Sum : Sum  Inputs=|+-
  Sum1 : Sum  Inputs=|++
  output : Outport
  wires:
  input/1 -> Delay/1, Sum/1
  Delay/1 -> Sum/2
  Sum/1 -> Sum1/1
  Sum1/1 -> Delay1/1, Gain/1
  Delay1/1 -> Sum1/2
  Gain/1 -> output/1

== system H8_2GDL_lineal_pruebas/Airgap Sensor3/Ruido ==
  Señal : Inport
  Random Number : RandomNumber  Mean=M  Variance=V  Seed=3  SampleTime=T
  Sum : Sum  Inputs=|++
  Señal_ruido : Outport
  wires:
  Random Number/1 -> Sum/2
  Señal/1 -> Sum/1
  Sum/1 -> Señal_ruido/1

== system H8_2GDL_lineal_pruebas/Airgap Sensor4/Discr_Ampl ==
  señal : Inport
  Constant : Constant  Value=N
  Constant1 : Constant  Value=Max
  Constant2 : Constant  Value=Min
  MATLAB Function1 : MATLAB Function  TreatAsAtomicUnit=on
  señal_discretizada : Outport
  wires:
  MATLAB Function1/1(senal_discretizada) -> señal_discretizada/1
  señal/1 -> MATLAB Function1/1(senal)
  Constant1/1 -> MATLAB Function1/3(Max)
  Constant/1 -> MATLAB Function1/2(N)
  Constant2/1 -> MATLAB Function1/4(Min)

== system H8_2GDL_lineal_pruebas/Airgap Sensor4/Moving Average Filter ==
  input : Inport
  Delay : Delay  DelayLength=M  SampleTime=fs
  Delay1 : Delay  DelayLength=1  SampleTime=fs
  Gain : Gain  Gain=1/M
  Sum : Sum  Inputs=|+-
  Sum1 : Sum  Inputs=|++
  output : Outport
  wires:
  input/1 -> Delay/1, Sum/1
  Delay/1 -> Sum/2
  Sum/1 -> Sum1/1
  Sum1/1 -> Delay1/1, Gain/1
  Delay1/1 -> Sum1/2
  Gain/1 -> output/1

== system H8_2GDL_lineal_pruebas/Airgap Sensor4/Ruido ==
  Señal : Inport
  Random Number : RandomNumber  Mean=M  Variance=V  Seed=3  SampleTime=T
  Sum : Sum  Inputs=|++
  Señal_ruido : Outport
  wires:
  Random Number/1 -> Sum/2
  Señal/1 -> Sum/1
  Sum/1 -> Señal_ruido/1

== system H8_2GDL_lineal_pruebas/RL/Subsystem ==
  Current : Inport
  Temperature : Inport  Port=2
  Resistance : Constant  Value=hems.Resistance
  R : Outport
  wires:
  Resistance/1 -> R/1

== system H8_2GDL_lineal_pruebas/RL1/Subsystem ==
  Current : Inport
  Temperature : Inport  Port=2
  Resistance : Constant  Value=hems.Resistance
  R : Outport
  wires:
  Resistance/1 -> R/1

== system H8_2GDL_lineal_pruebas/RL2/Subsystem ==
  Current : Inport
  Temperature : Inport  Port=2
  Resistance : Constant  Value=hems.Resistance
  R : Outport
  wires:
  Resistance/1 -> R/1

== system H8_2GDL_lineal_pruebas/RL3/Subsystem ==
  Current : Inport
  Temperature : Inport  Port=2
  Resistance : Constant  Value=hems.Resistance
  R : Outport
  wires:
  Resistance/1 -> R/1

== system H8_2GDL_lineal_pruebas/state-space control/Moving Average Filter ==
  input : Inport
  Delay : Delay  DelayLength=M  SampleTime=fs
  Delay1 : Delay  DelayLength=1  SampleTime=fs
  Gain : Gain  Gain=1/M
  Sum : Sum  Inputs=|+-
  Sum1 : Sum  Inputs=|++
  output : Outport
  wires:
  input/1 -> Delay/1, Sum/1
  Delay/1 -> Sum/2
  Sum/1 -> Sum1/1
  Sum1/1 -> Delay1/1, Gain/1
  Delay1/1 -> Sum1/2
  Gain/1 -> output/1

== system H8_2GDL_lineal_pruebas/state-space control/Moving Average Filter1 ==
  input : Inport
  Delay : Delay  DelayLength=M  SampleTime=fs
  Delay1 : Delay  DelayLength=1  SampleTime=fs
  Gain : Gain  Gain=1/M
  Sum : Sum  Inputs=|+-
  Sum1 : Sum  Inputs=|++
  output : Outport
  wires:
  input/1 -> Delay/1, Sum/1
  Delay/1 -> Sum/2
  Sum/1 -> Sum1/1
  Sum1/1 -> Delay1/1, Gain/1
  Delay1/1 -> Sum1/2
  Gain/1 -> output/1

== system H8_2GDL_lineal_pruebas/state-space control1/Moving Average Filter ==
  input : Inport
  Delay : Delay  DelayLength=M  SampleTime=fs
  Delay1 : Delay  DelayLength=1  SampleTime=fs
  Gain : Gain  Gain=1/M
  Sum : Sum  Inputs=|+-
  Sum1 : Sum  Inputs=|++
  output : Outport
  wires:
  input/1 -> Delay/1, Sum/1
  Delay/1 -> Sum/2
  Sum/1 -> Sum1/1
  Sum1/1 -> Delay1/1, Gain/1
  Delay1/1 -> Sum1/2
  Gain/1 -> output/1

== system H8_2GDL_lineal_pruebas/state-space control1/Moving Average Filter1 ==
  input : Inport
  Delay : Delay  DelayLength=M  SampleTime=fs
  Delay1 : Delay  DelayLength=1  SampleTime=fs
  Gain : Gain  Gain=1/M
  Sum : Sum  Inputs=|+-
  Sum1 : Sum  Inputs=|++
  output : Outport
  wires:
  input/1 -> Delay/1, Sum/1
  Delay/1 -> Sum/2
  Sum/1 -> Sum1/1
  Sum1/1 -> Delay1/1, Gain/1
  Delay1/1 -> Sum1/2
  Gain/1 -> output/1

== matlab function H8_2GDL_lineal_pruebas/Airgap Sensor1/Discr_Ampl/MATLAB Function1 ==
  data: senal input; senal_discretizada output; N input; Max input; Min input
function senal_discretizada  = fcn(senal,N,Max,Min)

if(senal>Max)
    senal_discretizada=Max;
    return
elseif(senal<Min)
    senal_discretizada=Min;
    return
end

valor_escalon=(Max-Min)/(N-1);
i=Min;
 while(i<Max)
    if(i+valor_escalon/2>senal)
        senal_discretizada=i;
        return
    end
    i=i+valor_escalon;
end

      senal_discretizada=Max;
end

== matlab function H8_2GDL_lineal_pruebas/Airgap Sensor2/Discr_Ampl/MATLAB Function1 ==
  data: senal input; senal_discretizada output; N input; Max input; Min input
function senal_discretizada  = fcn(senal,N,Max,Min)

if(senal>Max)
    senal_discretizada=Max;
    return
elseif(senal<Min)
    senal_discretizada=Min;
    return
end

valor_escalon=(Max-Min)/(N-1);
i=Min;
 while(i<Max)
    if(i+valor_escalon/2>senal)
        senal_discretizada=i;
        return
    end
    i=i+valor_escalon;
end

      senal_discretizada=Max;
end

== matlab function H8_2GDL_lineal_pruebas/Airgap Sensor3/Discr_Ampl/MATLAB Function1 ==
  data: senal input; senal_discretizada output; N input; Max input; Min input
function senal_discretizada  = fcn(senal,N,Max,Min)

if(senal>Max)
    senal_discretizada=Max;
    return
elseif(senal<Min)
    senal_discretizada=Min;
    return
end

valor_escalon=(Max-Min)/(N-1);
i=Min;
 while(i<Max)
    if(i+valor_escalon/2>senal)
        senal_discretizada=i;
        return
    end
    i=i+valor_escalon;
end

      senal_discretizada=Max;
end

== matlab function H8_2GDL_lineal_pruebas/Airgap Sensor4/Discr_Ampl/MATLAB Function1 ==
  data: senal input; senal_discretizada output; N input; Max input; Min input
function senal_discretizada  = fcn(senal,N,Max,Min)

if(senal>Max)
    senal_discretizada=Max;
    return
elseif(senal<Min)
    senal_discretizada=Min;
    return
end

valor_escalon=(Max-Min)/(N-1);
i=Min;
 while(i<Max)
    if(i+valor_escalon/2>senal)
        senal_discretizada=i;
        return
    end
    i=i+valor_escalon;
end

      senal_discretizada=Max;
end
